simulink model "sparrow_sim"  (R2022b)
settings: Solver=VariableStepAuto  StartTime=t0  StopTime=tmax  MaxStep=dt  RelTol=1e-3
values from neighbouring files (symbols this model uses):
  alpha0 = 0    [main.m]
  altitude = 0    [main.m]
  delta_max = 5*rad    (= 0.0872664625997)    [main.m]
  delta_min = 0*rad    (= 0)    [main.m]
  Vm = 700    [main.m]
libraries: aerolibatmos2 x1
settings Model: Creator=mitch  LastModifiedBy=mitchell
settings DataIOCC: ReturnWorkspaceOutputs=off

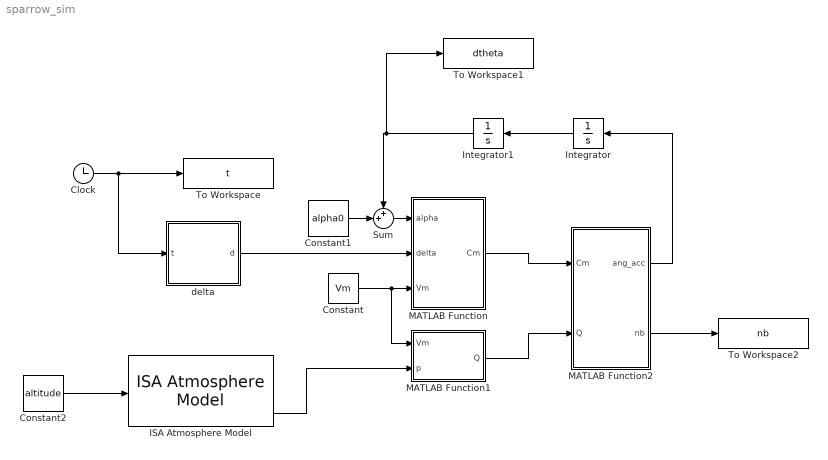
== system sparrow_sim ==
  Clock : Clock
  Constant : Constant  Value=Vm
  Constant1 : Constant  Value=alpha0
  Constant2 : Constant  Value=altitude
  ISA Atmosphere Model : aerolibatmos2/ISA Atmosphere Model  custom=off  g=9.80665  gamma=1.4  R=287.0531  L=0.0065  h_trop=11000  h_strat=20000  rho0=1.225  P0=101325  T0=288.15  h0=0
  Integrator : Integrator
  Integrator1 : Integrator
  MATLAB Function : MATLAB Function  TreatAsAtomicUnit=on
  MATLAB Function1 : MATLAB Function  TreatAsAtomicUnit=on
  MATLAB Function2 : MATLAB Function  TreatAsAtomicUnit=on
  Sum : Sum  Inputs=++|
  To Workspace : ToWorkspace  VariableName=t  SampleTime=-1
  To Workspace1 : ToWorkspace  VariableName=dtheta  SampleTime=-1
  To Workspace2 : ToWorkspace  VariableName=nb  SampleTime=-1
  delta : Subsystem
  wires:
  ISA Atmosphere Model/4 -> MATLAB Function1/2(p)
  Sum/1 -> MATLAB Function/1(alpha)
  Constant2/1 -> ISA Atmosphere Model/1
  Constant1/1 -> Sum/2
  MATLAB Function2/1(ang_acc) -> Integrator/1
  MATLAB Function1/1(Q) -> MATLAB Function2/2(Q)
  MATLAB Function2/2(nb) -> To Workspace2/1
  Clock/1 -> delta/1(t), To Workspace/1
  MATLAB Function/1(Cm) -> MATLAB Function2/1(Cm)
  Integrator1/1 -> To Workspace1/1, Sum/1
  delta/1(d) -> MATLAB Function/2(delta)
  Integrator/1 -> Integrator1/1
  Constant/1 -> MATLAB Function1/1(Vm), MATLAB Function/3(Vm)

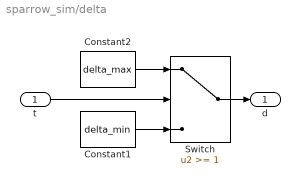
== system sparrow_sim/delta ==
  t : Inport
  Constant1 : Constant  Value=delta_min
  Constant2 : Constant  Value=delta_max
  Switch : Switch  Threshold=1  SaturateOnIntegerOverflow=off  InputSameDT=off
  d : Outport
  wires:
  t/1 -> Switch/2
  Switch/1 -> d/1
  Constant1/1 -> Switch/3
  Constant2/1 -> Switch/1

== matlab function sparrow_sim/MATLAB Function ==
  data: alpha input; Cm output; delta input; Vm input
function Cm = fcn(alpha, delta, Vm)

    %% Sparrow data

    L = 3.657;
    Ln = 0.193;
    d = 0.203;
    
    Xcg = 1.925;
    
    Crw = 0.495;
    Ctw = 0.097;
    Hw = 0.398;
    
    Crt = 0.473;
    Ctt = 0;
    Ht = 0.308;
    
    An = 0.67*Ln*d;
    Ab = (L-Ln)*d;
    
    Xhl = 1.829;
    
    %% Centers of pressure
    
    Xcpn = 0.67*Ln;
    Xcpb = ((0.67*An*Ln)+Ab*(Ln+0.5*(L-Ln)))/(An+Ab);
    Xcpt = L-0.3*Crt-0.2*Ctt;
    
    %% S values
    
    Sref = (pi*d^2)/4;
    Sw = 0.5*Hw*(Ctw+Crw);
    St = 0.5*Ht*(Ctt+Crt);
    Splan = ((L-Ln)*d)+(0.67*Ln*d);

    beta = sqrt(((Vm/343)^2)-1);

    Cm = ((2*alpha)*((Xcg-Xcpn)/d))+...
        (((1.5*Splan*alpha^2)/Sref)*((Xcg-Xcpb)/d))+...
        (((8*Sw*(alpha+delta))/(beta*Sref))*((Xcg-Xhl)/d))+...
        (((8*St*alpha)/(beta*Sref))*((Xcg-Xcpt)/d));

== matlab function sparrow_sim/MATLAB Function2 ==
  data: ang_acc output; Cm input; Q input; nb output
function [ang_acc, nb] = fcn(Cm, Q)

m = 120;
L = 3.657;
d = 0.203;

Sref = (pi*d^2)/4;
I = m*(3*((0.5*d)^2)+L^2);

nb = (Q*Sref*Cm)/m;
ang_acc = (Q*Sref*d*Cm)/I;

== matlab function sparrow_sim/MATLAB Function1 ==
  data: Vm input; p input; Q output
function Q = fcn(Vm, p)

Q = 0.5*p*Vm^2;
